simulink model "Correction_Simulation"  (R2024b)
settings: Solver=ode4  StartTime=0.0  StopTime=100  FixedStep=0.004  RelTol=1e-3
settings Model: Creator=leole  LastModifiedBy=leole

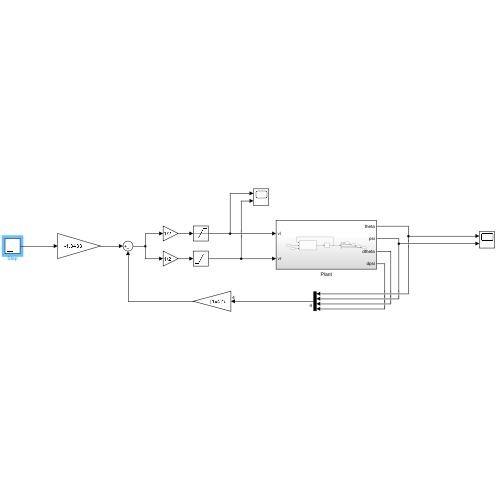
[thumbnail: Simulink's stored preview of the top-level diagram]
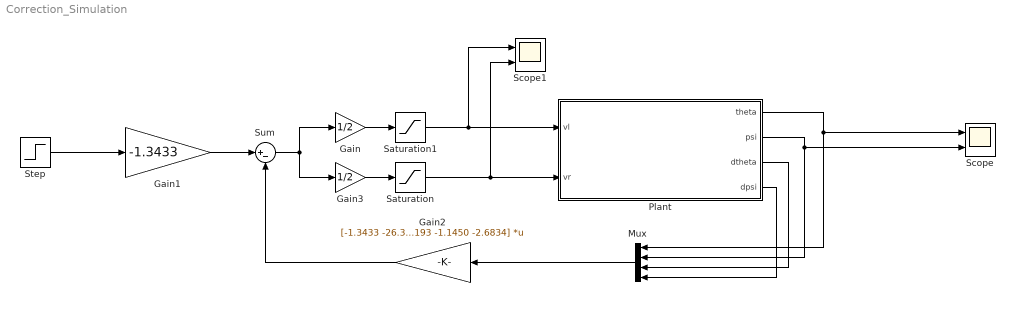
== system Correction_Simulation ==
  Gain : Gain  Gain=1/2
  Gain1 : Gain  Gain=-1.3433
  Gain2 : Gain  Gain=[-1.3433 -26.3193 -1.1450 -2.6834]  Multiplication=Matrix(K*u)
  Gain3 : Gain  Gain=1/2
  Mux : Mux
  Plant : Subsystem
  Saturation : Saturate  UpperLimit=8  LowerLimit=-8
  Saturation1 : Saturate  UpperLimit=8  LowerLimit=-8
  Scope : Scope  NumInputPorts=2
  Scope1 : Scope  NumInputPorts=2
  Step : Step  Time=20  After=10  SampleTime=0
  Sum : Sum  Inputs=|+-
  wires:
  Step/1 -> Gain1/1
  Gain1/1 -> Sum/1
  Gain2/1 -> Sum/2
  Plant/1(theta) -> Scope/1, Mux/1
  Plant/2(psi) -> Scope/2, Mux/2
  Plant/3(dtheta) -> Mux/3
  Plant/4(dpsi) -> Mux/4
  Mux/1 -> Gain2/1
  Sum/1 -> Gain3/1, Gain/1
  Gain3/1 -> Saturation/1
  Saturation/1 -> Scope1/2, Plant/2(vr)
  Gain/1 -> Saturation1/1
  Saturation1/1 -> Scope1/1, Plant/1(vl)

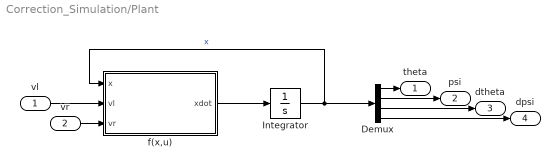
== system Correction_Simulation/Plant ==
  vl : Inport
  vr : Inport  Port=2
  Demux : Demux
  Integrator : Integrator  InitialCondition=[0; 0; 0; 0]
  f(x,u) : MATLAB Function  TreatAsAtomicUnit=on
  theta : Outport
  psi : Outport  Port=2
  dtheta : Outport  Port=3
  dpsi : Outport  Port=4
  wires:
  Integrator/1 -> f(x,u)/1(x), Demux/1  "x"
  f(x,u)/1(xdot) -> Integrator/1
  vl/1 -> f(x,u)/2(vl)
  Demux/1 -> theta/1
  Demux/2 -> psi/1
  Demux/3 -> dtheta/1
  Demux/4 -> dpsi/1
  vr/1 -> f(x,u)/3(vr)

== matlab function Correction_Simulation/Plant/f(x,u) ==
  data: x input; xdot output; vl input; vr input
function xdot =  compute_xdot(x, vl, vr)
%
% This function computes the x dot vector of the system (state derivative). It is used in
% the simulation simulink file to run the dynamical model of the
% gyropode.

% system parameters (defined in initialisation.m)
g = 9.80665;                    
m = 0.03;						
R = 0.042;						
Jw = m * R^2 / 2;				
M = 0.67;						
W = 0.165;						
D = 0.05;						
H = 0.152;						
L = H / 2;						
Jpsi = M * L^2 / 3;				
fm = 0.0022;					
fw = 0;								
Jm = 1e-5;						
Rm = 6.8327;					
Kb = 0.468;						
Kt = 0.3047;					
n = 1;
Jphi = M * (W^2 + D^2) / 12;

alpha = n * Kt / Rm;
beta = n * Kt * Kb / Rm + fm;

% position vector
theta = x(1);
psi = x(2);
% speed vector
dtheta = x(3);
dpsi = x(4);


Ftheta = 2*alpha*(vl+vr)-2*(beta+fw)*dtheta+2*beta*dpsi;

Fpsi = -2*alpha*(vl+vr)+2*beta*dtheta-2*beta*dpsi;

M1 = [ ((2*m+M)*R^2+2*Jw+2*n^2*Jm)  (M*L*R*cos(psi)-2*n^2*Jm);
       (M*L*R*cos(psi)-2*n^2*Jm)    (M*L^2+Jpsi+2*n^2*Jm)];
M2 = [ Ftheta+M*L*R*dpsi^2*sin(psi);
       Fpsi+M*g*L*sin(psi)];
var = M1\M2;

xdot1 = dtheta;
xdot2 = dpsi;
xdot3 = var(1);
xdot4 = var(2);

xdot = [xdot1;xdot2;xdot3;xdot4];
